simulink model "highpassfilter"  (R2020b)
settings: Solver=VariableStepAuto  StartTime=0.0  StopTime=10.0  RelTol=1e-3
settings Model: Creator=abhin  LastModifiedBy=abhin

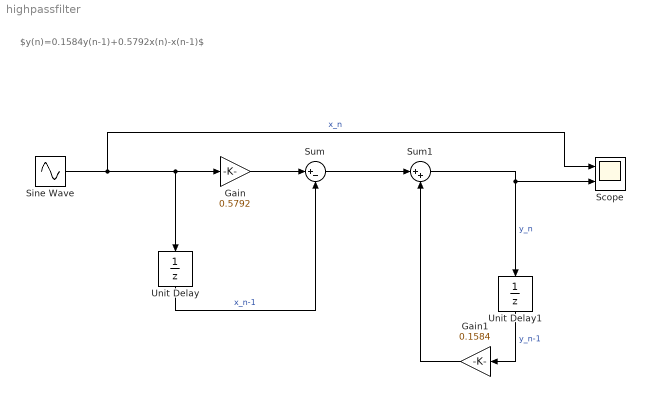
== system highpassfilter ==
  note: $y(n)=0.1584y(n-1)+0.5792x(n)-x(n-1)$
  Gain : Gain  Gain=0.5792
  Gain1 : Gain  Gain=0.1584
  Scope : Scope  NumInputPorts=2
  Sine Wave : Sin  Frequency=2*pi*200  SampleTime=0
  Sum : Sum  Inputs=|+-
  Sum1 : Sum  Inputs=|++
  Unit Delay : UnitDelay  SampleTime=-1  HasFrameUpgradeWarning=on
  Unit Delay1 : UnitDelay  SampleTime=-1  HasFrameUpgradeWarning=on
  wires:
  Sine Wave/1 -> Scope/1, Unit Delay/1, Gain/1  "x_n"
  Gain/1 -> Sum/1
  Unit Delay/1 -> Sum/2  "x_n-1"
  Sum/1 -> Sum1/1
  Sum1/1 -> Unit Delay1/1, Scope/2  "y_n"
  Unit Delay1/1 -> Gain1/1  "y_n-1"
  Gain1/1 -> Sum1/2
